simulink model "pratica10"  (R2021b)
settings: Solver=VariableStepAuto  StartTime=0.0  StopTime=24.00  RelTol=1e-3
values from neighbouring files (symbols this model uses):
  R = 1.15    [pratica10.m]
  T01 = (2*pi)/ws    [pratica10.m]
  T02 = 1.33*T01    [pratica10.m]
libraries: cstblocks x4
settings Model: Creator=carlo  LastModifiedBy=carlo

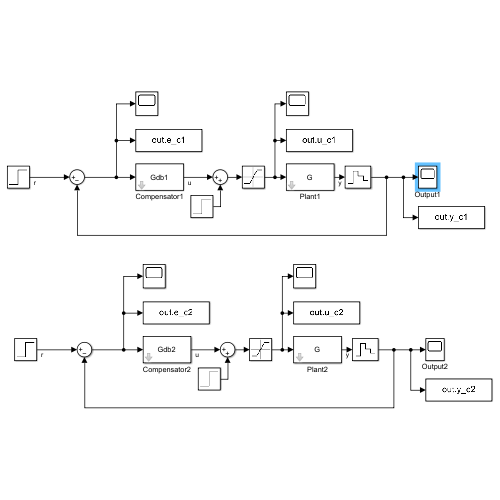
[thumbnail: Simulink's stored preview of the top-level diagram]
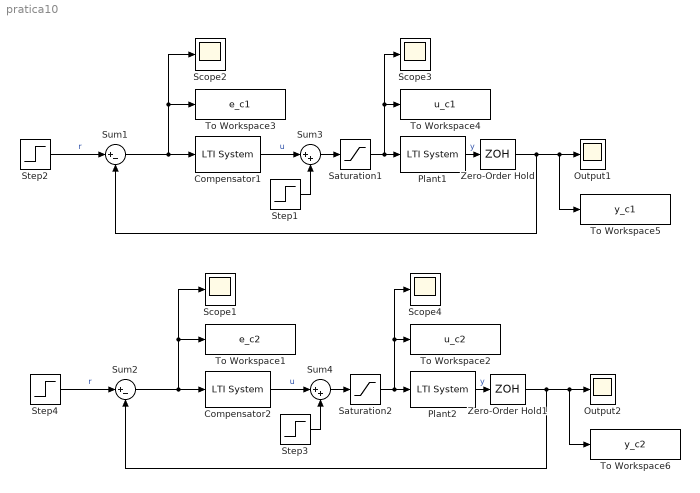
== system pratica10 ==
  Compensator1 : cstblocks/LTI System  sys=Gdb1  IC=[]
  Compensator2 : cstblocks/LTI System  sys=Gdb2  IC=[]
  Output1 : Scope
  Output2 : Scope
  Plant1 : cstblocks/LTI System  sys=G  IC=[]
  Plant2 : cstblocks/LTI System  sys=G  IC=[]
  Saturation1 : Saturate  UpperLimit=10  LowerLimit=-10
  Saturation2 : Saturate  UpperLimit=10  LowerLimit=-10
  Scope{1..4} (4 alike) : Scope
  Step1 : Step  Time=12  After=0.26  SampleTime=0
  Step2 : Step  Time=0  After=R  SampleTime=0
  Step3 : Step  Time=12  After=0.26  SampleTime=0
  Step4 : Step  Time=0  After=R  SampleTime=0
  Sum1 : Sum  Inputs=|+-
  Sum2 : Sum  Inputs=|+-
  Sum3 : Sum  Inputs=|++
  Sum4 : Sum  Inputs=|++
  To Workspace1 : ToWorkspace  VariableName=e_c2  SaveFormat=Timeseries  SampleTime=-1
  To Workspace2 : ToWorkspace  VariableName=u_c2  SaveFormat=Timeseries  SampleTime=-1
  To Workspace3 : ToWorkspace  VariableName=e_c1  SaveFormat=Timeseries  SampleTime=-1
  To Workspace4 : ToWorkspace  VariableName=u_c1  SaveFormat=Timeseries  SampleTime=-1
  To Workspace5 : ToWorkspace  VariableName=y_c1  SaveFormat=Timeseries  SampleTime=-1
  To Workspace6 : ToWorkspace  VariableName=y_c2  SaveFormat=Timeseries  SampleTime=-1
  Zero-Order Hold : ZeroOrderHold  SampleTime=T01
  Zero-Order Hold1 : ZeroOrderHold  SampleTime=T02
  wires:
  Step2/1 -> Sum1/1  "r"
  Step1/1 -> Sum3/2
  Sum1/1 -> Compensator1/1, To Workspace3/1, Scope2/1
  Sum3/1 -> Saturation1/1
  Plant1/1 -> Zero-Order Hold/1  "y"
  Saturation1/1 -> To Workspace4/1, Scope3/1, Plant1/1
  Compensator1/1 -> Sum3/1  "u"
  Zero-Order Hold/1 -> Sum1/2, To Workspace5/1, Output1/1
  Sum2/1 -> Compensator2/1, To Workspace1/1, Scope1/1
  Compensator2/1 -> Sum4/1  "u"
  Zero-Order Hold1/1 -> Sum2/2, To Workspace6/1, Output2/1
  Saturation2/1 -> To Workspace2/1, Scope4/1, Plant2/1
  Sum4/1 -> Saturation2/1
  Plant2/1 -> Zero-Order Hold1/1  "y"
  Step3/1 -> Sum4/2
  Step4/1 -> Sum2/1  "r"
